simulink model "ATV_sim"  (R2020b)
settings: Solver=VariableStepAuto  StartTime=0.0  StopTime=10.0  RelTol=1e-9
values from neighbouring files (symbols this model uses):
  Kc = 1000    [ATV.m]
  Kp = 2    [ATV.m]
  PD = [10 1]    [ATV.m]
  PDLY = 1    [ATV.m]
  PN = 1    [ATV.m]
settings Model: Creator=שקד  LastModifiedBy=Douaa
settings DataIOCC: ReturnWorkspaceOutputs=off

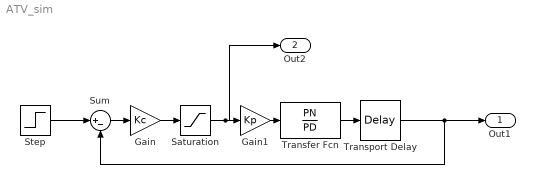
== system ATV_sim ==
  Gain : Gain  Gain=Kc
  Gain1 : Gain  Gain=Kp
  Saturation : Saturate  UpperLimit=1  LowerLimit=-1
  Step : Step  Time=0  After=1e-6  SampleTime=0
  Sum : Sum  Inputs=|+-
  Transfer Fcn : TransferFcn  Numerator=PN  Denominator=PD
  Transport Delay : TransportDelay  DelayTime=PDLY
  Out1 : Outport
  Out2 : Outport  Port=2
  wires:
  Transfer Fcn/1 -> Transport Delay/1
  Transport Delay/1 -> Sum/2, Out1/1
  Gain/1 -> Saturation/1
  Step/1 -> Sum/1
  Sum/1 -> Gain/1
  Saturation/1 -> Out2/1, Gain1/1
  Gain1/1 -> Transfer Fcn/1
